simulink library "Lib_LongPRACH"  (R2023b)
settings: Solver=VariableStepAuto  StartTime=0.0  StopTime=10.0  RelTol=1e-3
values from neighbouring files (symbols this model uses):
  prach = waveconfig.PRACH.Config    [hNRPRACHWaveformGenerator.m]
undefined symbols (not defined in the file or in its folder): AdvDSPBChannelOutDisplay, AdvDSPBDMemDisplay, AdvDSPBInDisplay, AdvDSPBOutDisplay, dpoly, dspba, dspba_ChannelInVis, dspba_ChannelOutVis, dspba_internal_get_channel_ports, evalAionMaskParam, latency, latencyCorrection, NTxAnts, primtype, UseDontCare, value
libraries: DSPBAPrim x553, DSPBABase x32, DSPBAFilters x24, DSPBAControl x18, DSPBAModelBus x8, DSPBAWaveformSynth x4, DspbAdvFftLibrary x2, DSPBAUtilities x2
(part 4 of 8)

== system Lib_LongPRACH/prach_wrap/DECIMATION/Filt_DEC_by_2_stage3 ==
  din : Inport
  vin : Inport  Port=2
  cin : Inport  Port=3
  Complex to Real-Imag : ComplexToRealImag
  Const1 : DSPBAPrim/Const  primtype=const  nInputs=0  nOutputs=1  omode=Inherit via back propagation  otype=ufix(8)  scale=2^0  rndmethod=Unbiased  factor=1  satmethod=Symmetric  shift_vec=[0 1 2 -1]  value=deimator_shift  inPortNames=['+'; '+';]  outPortNames=[' ']  dspbaimage=dspba_prim.svg  text=fprintf('%s', num2str(value));  style=Optimised  visibilities=8 + 1024  floatPrecision=float32_m23  warnSaturation=on  version=20211007  SampleTime=inf
  Const6 : DSPBAPrim/Const  primtype=const  nInputs=0  nOutputs=1  omode=Inherit via back propagation  otype=ufix(8)  scale=2^0  rndmethod=Unbiased  factor=1  satmethod=Symmetric  shift_vec=[0 1 2 -1]  value=deimator_shift  inPortNames=['+'; '+';]  outPortNames=[' ']  dspbaimage=dspba_prim.svg  text=fprintf('%s', num2str(value));  style=Optimised  visibilities=8 + 1024  floatPrecision=float32_m23  warnSaturation=on  version=20211007  SampleTime=inf
  DecimatingFIR : DSPBAFilters/DecimatingFIR  nInputRate=prach.MaxSampleRate/(3*2)  decim=2  nchan=prach.no_of_chan  symmetry=Symmetrical  coef=b_decimator3  addr=MMoffset.HBcoef3  rwmode=Constant  nband=Use All Taps  exposebus=off  latency=46  version=20090407  recon=off  MM=[0,1,2,3,4,5,6,7,8,9,10,11,12,13,14,15]  resetrezero=off  sharecoef=auto  simulationMode=Standard
  DecimatingFIR1 : DSPBAFilters/DecimatingFIR  nInputRate=prach.MaxSampleRate/(3*2)  decim=2  nchan=prach.no_of_chan  symmetry=Symmetrical  coef=b_decimator3  addr=MMoffset.HBcoef3  rwmode=Constant  nband=Use All Taps  exposebus=off  latency=46  version=20090407  recon=off  MM=[0,1,2,3,4,5,6,7,8,9,10,11,12,13,14,15]  resetrezero=off  sharecoef=auto  simulationMode=Standard
  Real-Imag to Complex : RealImagToComplex
  Scale : DSPBABase/Scale  otype=sfix(16)  scale=2^-15  rndmethod=Biased  factor=decimator_gain3  satmethod=Symmetric  shift_vec=0  latency=5  simulationMode=Use Global Value  version=20130807
  Scale1 : DSPBABase/Scale  otype=sfix(16)  scale=2^-15  rndmethod=Biased  factor=decimator_gain3  satmethod=Symmetric  shift_vec=0  latency=5  simulationMode=Use Global Value  version=20130807
  Terminator{,1..3} (4 alike) : Terminator
  To Workspace3 : ToWorkspace  VariableName=dec_dout_stage3  SampleTime=-1
  To Workspace4 : ToWorkspace  VariableName=dec_vout_stage3  SampleTime=-1
  dout : Outport  VectorParamsAs1DForOutWhenUnconnected=off
  vout : Outport  Port=2  VectorParamsAs1DForOutWhenUnconnected=off
  cout : Outport  Port=3  VectorParamsAs1DForOutWhenUnconnected=off
  wires:
  DecimatingFIR/1 -> Scale/1
  Const6/1 -> Scale/4
  cin/1 -> DecimatingFIR1/3, DecimatingFIR/3
  Scale/4 -> Terminator/1
  DecimatingFIR/3 -> Scale/3
  vin/1 -> DecimatingFIR1/2, DecimatingFIR/2
  DecimatingFIR/2 -> Scale/2
  Scale/3 -> cout/1
  din/1 -> Complex to Real-Imag/1
  Complex to Real-Imag/1 -> DecimatingFIR/1
  Complex to Real-Imag/2 -> DecimatingFIR1/1
  DecimatingFIR1/1 -> Scale1/1
  DecimatingFIR1/3 -> Scale1/3
  Scale1/1 -> Real-Imag to Complex/2
  DecimatingFIR1/2 -> Scale1/2
  Const1/1 -> Scale1/4
  Scale1/4 -> Terminator1/1
  Scale/1 -> Real-Imag to Complex/1
  Scale1/2 -> Terminator2/1
  Scale1/3 -> Terminator3/1
  Scale/2 -> To Workspace4/1, vout/1
  Real-Imag to Complex/1 -> To Workspace3/1, dout/1

== system Lib_LongPRACH/prach_wrap/DECIMATION/Filt_DEC_by_2_stage4 ==
  din : Inport
  vin : Inport  Port=2
  cin : Inport  Port=3
  Complex to Real-Imag : ComplexToRealImag
  Const1 : DSPBAPrim/Const  primtype=const  nInputs=0  nOutputs=1  omode=Inherit via back propagation  otype=ufix(8)  scale=2^0  rndmethod=Unbiased  factor=1  satmethod=Symmetric  shift_vec=[0 1 2 -1]  value=deimator_shift  inPortNames=['+'; '+';]  outPortNames=[' ']  dspbaimage=dspba_prim.svg  text=fprintf('%s', num2str(value));  style=Optimised  visibilities=8 + 1024  floatPrecision=float32_m23  warnSaturation=on  version=20211007  SampleTime=inf
  Const6 : DSPBAPrim/Const  primtype=const  nInputs=0  nOutputs=1  omode=Inherit via back propagation  otype=ufix(8)  scale=2^0  rndmethod=Unbiased  factor=1  satmethod=Symmetric  shift_vec=[0 1 2 -1]  value=deimator_shift  inPortNames=['+'; '+';]  outPortNames=[' ']  dspbaimage=dspba_prim.svg  text=fprintf('%s', num2str(value));  style=Optimised  visibilities=8 + 1024  floatPrecision=float32_m23  warnSaturation=on  version=20211007  SampleTime=inf
  DecimatingFIR : DSPBAFilters/DecimatingFIR  nInputRate=prach.MaxSampleRate/(3*2*2)  decim=2  nchan=prach.no_of_chan  symmetry=Symmetrical  coef=b_decimator4  addr=MMoffset.HBcoef3  rwmode=Constant  nband=Use All Taps  exposebus=off  latency=98  version=20090407  recon=off  MM=[0,1,2,3,4,5,6,7,8,9,10,11,12,13,14,15]  resetrezero=off  sharecoef=auto  simulationMode=Standard
  DecimatingFIR1 : DSPBAFilters/DecimatingFIR  nInputRate=prach.MaxSampleRate/(3*2*2)  decim=2  nchan=prach.no_of_chan  symmetry=Symmetrical  coef=b_decimator4  addr=MMoffset.HBcoef3  rwmode=Constant  nband=Use All Taps  exposebus=off  latency=98  version=20090407  recon=off  MM=[0,1,2,3,4,5,6,7,8,9,10,11,12,13,14,15]  resetrezero=off  sharecoef=auto  simulationMode=Standard
  Real-Imag to Complex : RealImagToComplex
  Scale : DSPBABase/Scale  otype=sfix(16)  scale=2^-15  rndmethod=Biased  factor=decimator_gain4  satmethod=Symmetric  shift_vec=0  latency=5  simulationMode=Use Global Value  version=20130807
  Scale1 : DSPBABase/Scale  otype=sfix(16)  scale=2^-15  rndmethod=Biased  factor=decimator_gain4  satmethod=Symmetric  shift_vec=0  latency=5  simulationMode=Use Global Value  version=20130807
  Terminator{,1..3} (4 alike) : Terminator
  To Workspace3 : ToWorkspace  VariableName=dec_dout_stage4  SampleTime=-1
  To Workspace4 : ToWorkspace  VariableName=dec_vout_stage4  SampleTime=-1
  dout : Outport  VectorParamsAs1DForOutWhenUnconnected=off
  vout : Outport  Port=2  VectorParamsAs1DForOutWhenUnconnected=off
  cout : Outport  Port=3  VectorParamsAs1DForOutWhenUnconnected=off
  wires:
  DecimatingFIR/1 -> Scale/1
  Const6/1 -> Scale/4
  cin/1 -> DecimatingFIR1/3, DecimatingFIR/3
  Scale/4 -> Terminator/1
  DecimatingFIR/3 -> Scale/3
  vin/1 -> DecimatingFIR1/2, DecimatingFIR/2
  DecimatingFIR/2 -> Scale/2
  Scale/3 -> cout/1
  din/1 -> Complex to Real-Imag/1
  Complex to Real-Imag/1 -> DecimatingFIR/1
  Complex to Real-Imag/2 -> DecimatingFIR1/1
  DecimatingFIR1/1 -> Scale1/1
  DecimatingFIR1/3 -> Scale1/3
  Scale1/1 -> Real-Imag to Complex/2
  DecimatingFIR1/2 -> Scale1/2
  Const1/1 -> Scale1/4
  Scale1/4 -> Terminator1/1
  Scale/1 -> Real-Imag to Complex/1
  Scale1/2 -> Terminator2/1
  Scale1/3 -> Terminator3/1
  Scale/2 -> To Workspace4/1, vout/1
  Real-Imag to Complex/1 -> To Workspace3/1, dout/1

== system Lib_LongPRACH/prach_wrap/DECIMATION/Filt_DEC_by_2_stage5 ==
  din : Inport
  vin : Inport  Port=2
  cin : Inport  Port=3
  Complex to Real-Imag : ComplexToRealImag
  Const1 : DSPBAPrim/Const  primtype=const  nInputs=0  nOutputs=1  omode=Inherit via back propagation  otype=ufix(8)  scale=2^0  rndmethod=Unbiased  factor=1  satmethod=Symmetric  shift_vec=[0 1 2 -1]  value=deimator_shift  inPortNames=['+'; '+';]  outPortNames=[' ']  dspbaimage=dspba_prim.svg  text=fprintf('%s', num2str(value));  style=Optimised  visibilities=8 + 1024  floatPrecision=float32_m23  warnSaturation=on  version=20211007  SampleTime=inf
  Const6 : DSPBAPrim/Const  primtype=const  nInputs=0  nOutputs=1  omode=Inherit via back propagation  otype=ufix(8)  scale=2^0  rndmethod=Unbiased  factor=1  satmethod=Symmetric  shift_vec=[0 1 2 -1]  value=deimator_shift  inPortNames=['+'; '+';]  outPortNames=[' ']  dspbaimage=dspba_prim.svg  text=fprintf('%s', num2str(value));  style=Optimised  visibilities=8 + 1024  floatPrecision=float32_m23  warnSaturation=on  version=20211007  SampleTime=inf
  DecimatingFIR : DSPBAFilters/DecimatingFIR  nInputRate=prach.MaxSampleRate/(3*2*2*2)  decim=2  nchan=prach.no_of_chan  symmetry=Symmetrical  coef=b_decimator5  addr=MMoffset.HBcoef3  rwmode=Constant  nband=Use All Taps  exposebus=off  latency=176  version=20090407  recon=off  MM=[0,1,2,3,4,5,6,7,8,9,10,11,12,13,14,15]  resetrezero=off  sharecoef=auto  simulationMode=Standard
  DecimatingFIR1 : DSPBAFilters/DecimatingFIR  nInputRate=prach.MaxSampleRate/(3*2*2*2)  decim=2  nchan=prach.no_of_chan  symmetry=Symmetrical  coef=b_decimator5  addr=MMoffset.HBcoef3  rwmode=Constant  nband=Use All Taps  exposebus=off  latency=176  version=20090407  recon=off  MM=[0,1,2,3,4,5,6,7,8,9,10,11,12,13,14,15]  resetrezero=off  sharecoef=auto  simulationMode=Standard
  Real-Imag to Complex : RealImagToComplex
  Scale : DSPBABase/Scale  otype=sfix(16)  scale=2^-15  rndmethod=Biased  factor=decimator_gain5  satmethod=Symmetric  shift_vec=0  latency=5  simulationMode=Use Global Value  version=20130807
  Scale1 : DSPBABase/Scale  otype=sfix(16)  scale=2^-15  rndmethod=Biased  factor=decimator_gain5  satmethod=Symmetric  shift_vec=0  latency=5  simulationMode=Use Global Value  version=20130807
  Terminator{,1..3} (4 alike) : Terminator
  To Workspace3 : ToWorkspace  VariableName=dec_dout_stage5  SampleTime=-1
  To Workspace4 : ToWorkspace  VariableName=dec_vout_stage5  SampleTime=-1
  dout : Outport  VectorParamsAs1DForOutWhenUnconnected=off
  vout : Outport  Port=2  VectorParamsAs1DForOutWhenUnconnected=off
  cout : Outport  Port=3  VectorParamsAs1DForOutWhenUnconnected=off
  wires:
  DecimatingFIR/1 -> Scale/1
  Const6/1 -> Scale/4
  cin/1 -> DecimatingFIR1/3, DecimatingFIR/3
  Scale/4 -> Terminator/1
  DecimatingFIR/3 -> Scale/3
  vin/1 -> DecimatingFIR1/2, DecimatingFIR/2
  DecimatingFIR/2 -> Scale/2
  Scale/3 -> cout/1
  din/1 -> Complex to Real-Imag/1
  Complex to Real-Imag/1 -> DecimatingFIR/1
  Complex to Real-Imag/2 -> DecimatingFIR1/1
  DecimatingFIR1/1 -> Scale1/1
  DecimatingFIR1/3 -> Scale1/3
  Scale1/1 -> Real-Imag to Complex/2
  DecimatingFIR1/2 -> Scale1/2
  Const1/1 -> Scale1/4
  Scale1/4 -> Terminator1/1
  Scale/1 -> Real-Imag to Complex/1
  Scale1/2 -> Terminator2/1
  Scale1/3 -> Terminator3/1
  Scale/2 -> vout/1, To Workspace4/1
  Real-Imag to Complex/1 -> dout/1, To Workspace3/1

== system Lib_LongPRACH/prach_wrap/DECIMATION/Filt_DEC_by_2_stage6 ==
  din : Inport
  vin : Inport  Port=2
  cin : Inport  Port=3
  Complex to Real-Imag : ComplexToRealImag
  Const1 : DSPBAPrim/Const  primtype=const  nInputs=0  nOutputs=1  omode=Inherit via back propagation  otype=ufix(8)  scale=2^0  rndmethod=Unbiased  factor=1  satmethod=Symmetric  shift_vec=[0 1 2 -1]  value=deimator_shift  inPortNames=['+'; '+';]  outPortNames=[' ']  dspbaimage=dspba_prim.svg  text=fprintf('%s', num2str(value));  style=Optimised  visibilities=8 + 1024  floatPrecision=float32_m23  warnSaturation=on  version=20211007  SampleTime=inf
  Const6 : DSPBAPrim/Const  primtype=const  nInputs=0  nOutputs=1  omode=Inherit via back propagation  otype=ufix(8)  scale=2^0  rndmethod=Unbiased  factor=1  satmethod=Symmetric  shift_vec=[0 1 2 -1]  value=deimator_shift  inPortNames=['+'; '+';]  outPortNames=[' ']  dspbaimage=dspba_prim.svg  text=fprintf('%s', num2str(value));  style=Optimised  visibilities=8 + 1024  floatPrecision=float32_m23  warnSaturation=on  version=20211007  SampleTime=inf
  DecimatingFIR : DSPBAFilters/DecimatingFIR  nInputRate=prach.MaxSampleRate/(3*2*2*2*2)  decim=2  nchan=prach.no_of_chan  symmetry=Symmetrical  coef=b_decimator6  addr=MMoffset.HBcoef3  rwmode=Constant  nband=Use All Taps  exposebus=off  latency=208  version=20090407  recon=off  MM=[0,1,2,3,4,5,6,7,8,9,10,11,12,13,14,15]  resetrezero=off  sharecoef=auto  simulationMode=Standard
  DecimatingFIR1 : DSPBAFilters/DecimatingFIR  nInputRate=prach.MaxSampleRate/(3*2*2*2*2)  decim=2  nchan=prach.no_of_chan  symmetry=Symmetrical  coef=b_decimator6  addr=MMoffset.HBcoef3  rwmode=Constant  nband=Use All Taps  exposebus=off  latency=208  version=20090407  recon=off  MM=[0,1,2,3,4,5,6,7,8,9,10,11,12,13,14,15]  resetrezero=off  sharecoef=auto  simulationMode=Standard
  Real-Imag to Complex : RealImagToComplex
  Scale : DSPBABase/Scale  otype=sfix(16)  scale=2^-15  rndmethod=Biased  factor=decimator_gain6  satmethod=Symmetric  shift_vec=0  latency=5  simulationMode=Use Global Value  version=20130807
  Scale1 : DSPBABase/Scale  otype=sfix(16)  scale=2^-15  rndmethod=Biased  factor=decimator_gain6  satmethod=Symmetric  shift_vec=0  latency=5  simulationMode=Use Global Value  version=20130807
  Terminator{,1..3} (4 alike) : Terminator
  dout : Outport  VectorParamsAs1DForOutWhenUnconnected=off
  vout : Outport  Port=2  VectorParamsAs1DForOutWhenUnconnected=off
  cout : Outport  Port=3  VectorParamsAs1DForOutWhenUnconnected=off
  wires:
  DecimatingFIR/1 -> Scale/1
  Const6/1 -> Scale/4
  cin/1 -> DecimatingFIR1/3, DecimatingFIR/3
  Scale/4 -> Terminator/1
  Scale/2 -> vout/1
  DecimatingFIR/3 -> Scale/3
  vin/1 -> DecimatingFIR1/2, DecimatingFIR/2
  DecimatingFIR/2 -> Scale/2
  Scale/3 -> cout/1
  din/1 -> Complex to Real-Imag/1
  Complex to Real-Imag/1 -> DecimatingFIR/1
  Complex to Real-Imag/2 -> DecimatingFIR1/1
  DecimatingFIR1/1 -> Scale1/1
  DecimatingFIR1/3 -> Scale1/3
  Scale1/1 -> Real-Imag to Complex/2
  DecimatingFIR1/2 -> Scale1/2
  Const1/1 -> Scale1/4
  Scale1/4 -> Terminator1/1
  Scale/1 -> Real-Imag to Complex/1
  Real-Imag to Complex/1 -> dout/1
  Scale1/2 -> Terminator2/1
  Scale1/3 -> Terminator3/1

== system Lib_LongPRACH/prach_wrap/DECIMATION/Filt_DEC_by_3_stage1 ==
  din : Inport
  vin : Inport  Port=2
  cin : Inport  Port=3
  Complex to Real-Imag : ComplexToRealImag
  Const1 : DSPBAPrim/Const  primtype=const  nInputs=0  nOutputs=1  omode=Inherit via back propagation  otype=ufix(8)  scale=2^0  rndmethod=Unbiased  factor=1  satmethod=Symmetric  shift_vec=[0 1 2 -1]  value=deimator_shift  inPortNames=['+'; '+';]  outPortNames=[' ']  dspbaimage=dspba_prim.svg  text=fprintf('%s', num2str(value));  style=Optimised  visibilities=8 + 1024  floatPrecision=float32_m23  warnSaturation=on  version=20211007  SampleTime=inf
  Const6 : DSPBAPrim/Const  primtype=const  nInputs=0  nOutputs=1  omode=Inherit via back propagation  otype=ufix(8)  scale=2^0  rndmethod=Unbiased  factor=1  satmethod=Symmetric  shift_vec=[0 1 2 -1]  value=deimator_shift  inPortNames=['+'; '+';]  outPortNames=[' ']  dspbaimage=dspba_prim.svg  text=fprintf('%s', num2str(value));  style=Optimised  visibilities=8 + 1024  floatPrecision=float32_m23  warnSaturation=on  version=20211007  SampleTime=inf
  DecimatingFIR1 : DSPBAFilters/DecimatingFIR  nInputRate=prach.MaxSampleRate  decim=3  nchan=prach.no_of_chan  symmetry=Symmetrical  coef=b_decimator1  addr=MMoffset.decby3_st2  rwmode=Constant  nband=Use All Taps  exposebus=off  latency=26  version=20090407  recon=off  MM=[0,1,2,3,4,5,6,7,8,9,10,11,12,13,14,15]  resetrezero=off  sharecoef=auto  simulationMode=Standard
  DecimatingFIR2 : DSPBAFilters/DecimatingFIR  nInputRate=prach.MaxSampleRate  decim=3  nchan=prach.no_of_chan  symmetry=Symmetrical  coef=b_decimator1  addr=MMoffset.decby3_st2  rwmode=Constant  nband=Use All Taps  exposebus=off  latency=26  version=20090407  recon=off  MM=[0,1,2,3,4,5,6,7,8,9,10,11,12,13,14,15]  resetrezero=off  sharecoef=auto  simulationMode=Standard
  Real-Imag to Complex : RealImagToComplex
  Scale : DSPBABase/Scale  otype=sfix(16)  scale=2^-15  rndmethod=Biased  factor=decimator_gain1  satmethod=Symmetric  shift_vec=0  latency=5  simulationMode=Use Global Value  version=20130807
  Scale1 : DSPBABase/Scale  otype=sfix(16)  scale=2^-15  rndmethod=Biased  factor=decimator_gain1  satmethod=Symmetric  shift_vec=0  latency=5  simulationMode=Use Global Value  version=20130807
  Terminator : Terminator
  Terminator1 : Terminator
  To Workspace3 : ToWorkspace  VariableName=dec_dout_stage1  SampleTime=-1
  To Workspace4 : ToWorkspace  VariableName=dec_vout_stage1  SampleTime=-1
  dout : Outport  VectorParamsAs1DForOutWhenUnconnected=off
  vout : Outport  Port=2  VectorParamsAs1DForOutWhenUnconnected=off
  cout : Outport  Port=3  VectorParamsAs1DForOutWhenUnconnected=off
  wires:
  Scale/3 -> cout/1
  DecimatingFIR2/2 -> Scale/2
  vin/1 -> DecimatingFIR1/2, DecimatingFIR2/2
  DecimatingFIR2/3 -> Scale/3
  Scale/2 -> To Workspace4/1, vout/1
  Scale/4 -> Terminator/1
  cin/1 -> DecimatingFIR1/3, DecimatingFIR2/3
  Const6/1 -> Scale/4
  DecimatingFIR2/1 -> Scale/1
  din/1 -> Complex to Real-Imag/1
  Complex to Real-Imag/1 -> DecimatingFIR2/1
  Complex to Real-Imag/2 -> DecimatingFIR1/1
  Scale1/1 -> Real-Imag to Complex/2
  DecimatingFIR1/3 -> Scale1/3
  Scale1/4 -> Terminator1/1
  DecimatingFIR1/1 -> Scale1/1
  DecimatingFIR1/2 -> Scale1/2
  Const1/1 -> Scale1/4
  Real-Imag to Complex/1 -> To Workspace3/1, dout/1
  Scale/1 -> Real-Imag to Complex/1

== system Lib_LongPRACH/prach_wrap/FFTShift/ChNoLatch ==
  valid1 : Inport
  din : Inport  Port=2
  valid2 : Inport  Port=3
  FIFO : DSPBAPrim/FIFO  primtype=fifo  nInputs=3  nOutputs=4  omode=Inherit via internal rule  otype=sfix(16)  scale=2^-15  rndmethod=Unbiased  factor=1  satmethod=Symmetric  shift_vec=[0 1 2 -1]  value=[32 4 16]  inPortNames=['w'; 'd'; 'r'; 'f']  outPortNames=['v'; 'q'; 't'; 'f']  dspbaimage=dspba_prim_tall.svg  text=fprintf('fifo');  style=Optimised  visibilities=263168  version=20211007  user_sclr=off
  Terminator1 : Terminator
  Terminator2 : Terminator
  Terminator3 : Terminator
  risingedge : Subsystem
  risingedge1 : Subsystem
  dout : Outport
  wires:
  FIFO/3 -> Terminator1/1
  FIFO/1 -> Terminator3/1
  risingedge1/1(Out1) -> FIFO/3
  FIFO/4 -> Terminator2/1
  risingedge/1(Out1) -> FIFO/1
  valid2/1 -> risingedge1/1(In2)
  FIFO/2 -> dout/1
  valid1/1 -> risingedge/1(In2)
  din/1 -> FIFO/2

== system Lib_LongPRACH/prach_wrap/FFTShift/Mem_rd_wr ==
  valid : Inport
  Mem_rd_control : Subsystem
  Mem_wr_control : Subsystem
  Wr_addr_final : Outport
  We : Outport  Port=2
  rd_addr_final : Outport  Port=3
  rd_validout : Outport  Port=4
  wba : Outport  Port=5
  wires:
  valid/1 -> Mem_wr_control/1(valid)
  Mem_wr_control/1(wr_addr_final) -> Wr_addr_final/1
  Mem_wr_control/2(we) -> We/1
  Mem_wr_control/3(wba) -> wba/1, Mem_rd_control/1(wba)
  Mem_rd_control/1(rd_addr_final) -> rd_addr_final/1
  Mem_rd_control/2(validout) -> rd_validout/1

== system Lib_LongPRACH/prach_wrap/FFTShift/Subsystem ==
  toggleline : Inport
  d : Inport  Port=2
  SampleDelay : DSPBAPrim/SampleDelay  primtype=sampdelay  nInputs=1  nOutputs=1  omode=Inherit via internal rule  otype=sfix(16)  scale=2^-15  rndmethod=Unbiased  factor=1  satmethod=Symmetric  shift_vec=[0 1 2 -1]  floatPrecision=float32_m23  value=1  inPortNames=[' '; ' ';]  outPortNames=[' ']  dspbaimage=dspba_prim.svg  text=dpoly(1, eye(1,value+1), 'z')  style=Optimised  visibilities=8 + 2^11 + 2^18 + 2^19  flexible=off  slackgroup=0  augmented=0  version=20211007  advOptions=[]
  Xor : DSPBAPrim/Xor  primtype=xor  nInputs=2  nOutputs=1  omode=Inherit via internal rule  otype=sfix(16)  scale=2^-15  rndmethod=Unbiased  factor=1  satmethod=Symmetric  shift_vec=[0 1 2 -1]  value=0  inPortNames=[' '; ' '; ' '; ' '; ' '; ' '; ' '; ' '; ' '; ' '; ' '; ' '; ' '; ' '; ' '; ' '; ]  outPortNames=[' ']  dspbaimage=dspba_prim.svg  text=fprintf('^');  style=Optimised  visibilities=8+2  version=20211007
  latch_0L : DSPBAControl/latch_0L
  q : Outport
  wires:
  SampleDelay/1 -> Xor/1
  Xor/1 -> latch_0L/1
  latch_0L/1 -> q/1
  d/1 -> latch_0L/2
  toggleline/1 -> SampleDelay/1, Xor/2

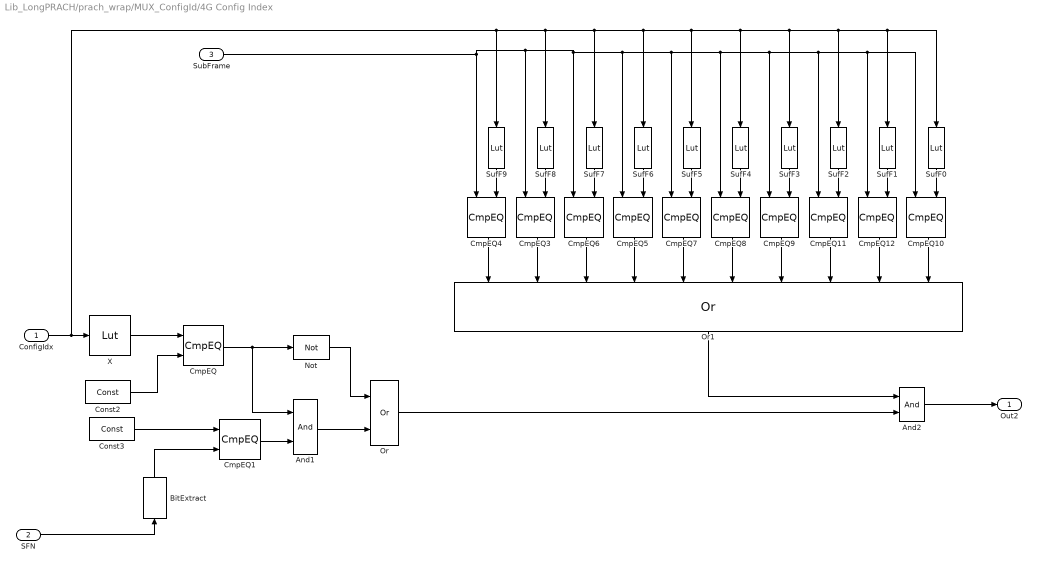
== system Lib_LongPRACH/prach_wrap/MUX_ConfigId/4G Config Index ==
  ConfigIdx : Inport
  SFN : Inport  Port=2
  SubFrame : Inport  Port=3
  And1 : DSPBAPrim/And  primtype=and  nInputs=2  nOutputs=1  omode=Inherit via internal rule  otype=sfix(16)  scale=2^-15  rndmethod=Unbiased  factor=1  satmethod=Symmetric  shift_vec=[0 1 2 -1]  value=0  inPortNames=[' '; ' '; ' '; ' '; ' '; ' '; ' '; ' '; ' '; ' '; ' '; ' '; ' '; ' '; ' '; ' '; ]  outPortNames=[' ']  dspbaimage=dspba_prim.svg  text=fprintf('&');  style=Optimised  visibilities=8+2  version=20211007
  And2 : DSPBAPrim/And  primtype=and  nInputs=2  nOutputs=1  omode=Inherit via internal rule  otype=sfix(16)  scale=2^-15  rndmethod=Unbiased  factor=1  satmethod=Symmetric  shift_vec=[0 1 2 -1]  value=0  inPortNames=[' '; ' '; ' '; ' '; ' '; ' '; ' '; ' '; ' '; ' '; ' '; ' '; ' '; ' '; ' '; ' '; ]  outPortNames=[' ']  dspbaimage=dspba_prim.svg  text=fprintf('&');  style=Optimised  visibilities=8+2  version=20211007
  BitExtract : DSPBAPrim/BitExtract  primtype=bitextract  nInputs=1  nOutputs=1  omode=Specify via dialog  otype=ufix(1)  scale=1  rndmethod=Unbiased  factor=1  satmethod=Symmetric  shift_vec=[0 1 2 -1]  value=0  inPortNames=[' '; ' ';]  outPortNames=[' ']  dspbaimage=dspba_prim.svg  text=fprintf('..%d', value);  style=Optimised  visibilities=8+1024  version=20211007
  CmpEQ{,1,3..12} (12 alike) : DSPBAPrim/CmpEQ  primtype=cmpeq  nInputs=2  nOutputs=1  omode=boolean  otype=sfix(16)  scale=2^-15  rndmethod=Unbiased  factor=1  satmethod=Symmetric  shift_vec=[0 1 2 -1]  value=0  inPortNames=[' '; ' ';]  outPortNames=[' ']  dspbaimage=dspba_prim.svg  text=fprintf('==');  style=Optimised  visibilities=0  advOptions=[]  version=20211007
  Const2 : DSPBAPrim/Const  primtype=const  nInputs=0  nOutputs=1  omode=Specify via dialog  otype=ufix(1)  scale=2^-0  rndmethod=Unbiased  factor=1  satmethod=Symmetric  shift_vec=[0 1 2 -1]  value=0  inPortNames=['+'; '+';]  outPortNames=[' ']  dspbaimage=dspba_prim.svg  text=fprintf('%s', num2str(value));  style=Optimised  visibilities=8 + 1024  floatPrecision=float32_m23  warnSaturation=on  version=20211007  SampleTime=inf
  Const3 : DSPBAPrim/Const  primtype=const  nInputs=0  nOutputs=1  omode=Specify via dialog  otype=ufix(1)  scale=2^-0  rndmethod=Unbiased  factor=1  satmethod=Symmetric  shift_vec=[0 1 2 -1]  value=0  inPortNames=['+'; '+';]  outPortNames=[' ']  dspbaimage=dspba_prim.svg  text=fprintf('%s', num2str(value));  style=Optimised  visibilities=8 + 1024  floatPrecision=float32_m23  warnSaturation=on  version=20211007  SampleTime=inf
  Not : DSPBAPrim/Not  primtype=not  nInputs=1  nOutputs=1  omode=Inherit via internal rule  otype=sfix(16)  scale=2^-15  rndmethod=Unbiased  factor=1  satmethod=Symmetric  shift_vec=[0 1 2 -1]  value=0  inPortNames=[' '; ' ';]  outPortNames=[' ']  dspbaimage=dspba_prim.svg  text=fprintf('~');  style=Optimised  visibilities=8  version=20211007
  Or : DSPBAPrim/Or  primtype=or  nInputs=2  nOutputs=1  omode=Inherit via internal rule  otype=sfix(16)  scale=2^-15  rndmethod=Unbiased  factor=1  satmethod=Symmetric  shift_vec=[0 1 2 -1]  value=0  inPortNames=[' '; ' '; ' '; ' '; ' '; ' '; ' '; ' '; ' '; ' '; ' '; ' '; ' '; ' '; ' '; ' '; ]  outPortNames=[' ']  dspbaimage=dspba_prim.svg  text=fprintf('|');  style=Optimised  visibilities=8+2  version=20211007
  Or1 : DSPBAPrim/Or  primtype=or  nInputs=10  nOutputs=1  omode=Inherit via internal rule  otype=sfix(16)  scale=2^-15  rndmethod=Unbiased  factor=1  satmethod=Symmetric  shift_vec=[0 1 2 -1]  value=0  inPortNames=[' '; ' '; ' '; ' '; ' '; ' '; ' '; ' '; ' '; ' '; ' '; ' '; ' '; ' '; ' '; ' '; ]  outPortNames=[' ']  dspbaimage=dspba_prim.svg  text=fprintf('|');  style=Optimised  visibilities=8+2  version=20211007
  SufF0 : DSPBAPrim/Lut  primtype=lut  nInputs=1  nOutputs=1  omode=Inherit via internal rule  otype=sfix(16)  scale=2^-15  rndmethod=Unbiased  factor=1  satmethod=Symmetric  shift_vec=[0 1 2 -1]  value=[1 4 7 1 4 7 1 2 3 1 2 3 0 1 0 9 zeros(1,256-16)]  inPortNames=[' '; ' ';]  outPortNames=[' ']  dspbaimage=dspba_prim.svg  text=fprintf('LUT');  style=Optimised  visibilities=8 + 1024  floatPrecision=float32_m23  version=20211007
  SufF1 : DSPBAPrim/Lut  primtype=lut  nInputs=1  nOutputs=1  omode=Inherit via internal rule  otype=sfix(16)  scale=2^-15  rndmethod=Unbiased  factor=1  satmethod=Symmetric  shift_vec=[0 1 2 -1]  value=[1 4 7 1 4 7 6 7 8 4 5 6 2 3 1 9 zeros(1,256-16)]  inPortNames=[' '; ' ';]  outPortNames=[' ']  dspbaimage=dspba_prim.svg  text=fprintf('LUT');  style=Optimised  visibilities=8 + 1024  floatPrecision=float32_m23  version=20211007
  SufF2 : DSPBAPrim/Lut  primtype=lut  nInputs=1  nOutputs=1  omode=Inherit via internal rule  otype=sfix(16)  scale=2^-15  rndmethod=Unbiased  factor=1  satmethod=Symmetric  shift_vec=[0 1 2 -1]  value=[1 4 7 1 4 7 6 7 8 7 8 9 4 5 2 9 zeros(1,256-16)]  inPortNames=[' '; ' ';]  outPortNames=[' ']  dspbaimage=dspba_prim.svg  text=fprintf('LUT');  style=Optimised  visibilities=8 + 1024  floatPrecision=float32_m23  version=20211007
  SufF3 : DSPBAPrim/Lut  primtype=lut  nInputs=1  nOutputs=1  omode=Inherit via internal rule  otype=sfix(16)  scale=2^-15  rndmethod=Unbiased  factor=1  satmethod=Symmetric  shift_vec=[0 1 2 -1]  value=[1 4 7 1 4 7 6 7 8 7 8 9 6 7 3 9 zeros(1,256-16)]  inPortNames=[' '; ' ';]  outPortNames=[' ']  dspbaimage=dspba_prim.svg  text=fprintf('LUT');  style=Optimised  visibilities=8 + 1024  floatPrecision=float32_m23  version=20211007
  SufF4 : DSPBAPrim/Lut  primtype=lut  nInputs=1  nOutputs=1  omode=Inherit via internal rule  otype=sfix(16)  scale=2^-15  rndmethod=Unbiased  factor=1  satmethod=Symmetric  shift_vec=[0 1 2 -1]  value=[1 4 7 1 4 7 6 7 8 7 8 9 8 9 4 9 zeros(1,256-16)]  inPortNames=[' '; ' ';]  outPortNames=[' ']  dspbaimage=dspba_prim.svg  text=fprintf('LUT');  style=Optimised  visibilities=8 + 1024  floatPrecision=float32_m23  version=20211007
  SufF5 : DSPBAPrim/Lut  primtype=lut  nInputs=1  nOutputs=1  omode=Inherit via internal rule  otype=sfix(16)  scale=2^-15  rndmethod=Unbiased  factor=1  satmethod=Symmetric  shift_vec=[0 1 2 -1]  value=[1 4 7 1 4 7 6 7 8 7 8 9 8 9 5 9 zeros(1,256-16)]  inPortNames=[' '; ' ';]  outPortNames=[' ']  dspbaimage=dspba_prim.svg  text=fprintf('LUT');  style=Optimised  visibilities=8 + 1024  floatPrecision=float32_m23  version=20211007
  SufF6 : DSPBAPrim/Lut  primtype=lut  nInputs=1  nOutputs=1  omode=Inherit via internal rule  otype=sfix(16)  scale=2^-15  rndmethod=Unbiased  factor=1  satmethod=Symmetric  shift_vec=[0 1 2 -1]  value=[1 4 7 1 4 7 6 7 8 7 8 9 8 9 6 9 zeros(1,256-16)]  inPortNames=[' '; ' ';]  outPortNames=[' ']  dspbaimage=dspba_prim.svg  text=fprintf('LUT');  style=Optimised  visibilities=8 + 1024  floatPrecision=float32_m23  version=20211007
  SufF7 : DSPBAPrim/Lut  primtype=lut  nInputs=1  nOutputs=1  omode=Inherit via internal rule  otype=sfix(16)  scale=2^-15  rndmethod=Unbiased  factor=1  satmethod=Symmetric  shift_vec=[0 1 2 -1]  value=[1 4 7 1 4 7 6 7 8 7 8 9 8 9 7 9 zeros(1,256-16)]  inPortNames=[' '; ' ';]  outPortNames=[' ']  dspbaimage=dspba_prim.svg  text=fprintf('LUT');  style=Optimised  visibilities=8 + 1024  floatPrecision=float32_m23  version=20211007
  SufF8 : DSPBAPrim/Lut  primtype=lut  nInputs=1  nOutputs=1  omode=Inherit via internal rule  otype=sfix(16)  scale=2^-15  rndmethod=Unbiased  factor=1  satmethod=Symmetric  shift_vec=[0 1 2 -1]  value=[1 4 7 1 4 7 6 7 8 7 8 9 8 9 8 9 zeros(1,256-16)]  inPortNames=[' '; ' ';]  outPortNames=[' ']  dspbaimage=dspba_prim.svg  text=fprintf('LUT');  style=Optimised  visibilities=8 + 1024  floatPrecision=float32_m23  version=20211007
  SufF9 : DSPBAPrim/Lut  primtype=lut  nInputs=1  nOutputs=1  omode=Inherit via internal rule  otype=sfix(16)  scale=2^-15  rndmethod=Unbiased  factor=1  satmethod=Symmetric  shift_vec=[0 1 2 -1]  value=[1 4 7 1 4 7 6 7 8 7 8 9 8 9 9 9 zeros(1,256-16)]  inPortNames=[' '; ' ';]  outPortNames=[' ']  dspbaimage=dspba_prim.svg  text=fprintf('LUT');  style=Optimised  visibilities=8 + 1024  floatPrecision=float32_m23  version=20211007
  X : DSPBAPrim/Lut  primtype=lut  nInputs=1  nOutputs=1  omode=Inherit via internal rule  otype=sfix(16)  scale=2^-15  rndmethod=Unbiased  factor=1  satmethod=Symmetric  shift_vec=[0 1 2 -1]  value=[0,0,0,1,1,1,1,1,1,1,1,1,1,1,1,0,ones(1,256-16)]  inPortNames=[' '; ' ';]  outPortNames=[' ']  dspbaimage=dspba_prim.svg  text=fprintf('LUT');  style=Optimised  visibilities=8 + 1024  floatPrecision=float32_m23  version=20211007
  Out2 : Outport
  wires:
  Const3/1 -> CmpEQ1/1
  CmpEQ/1 -> Not/1, And1/1
  CmpEQ1/1 -> And1/2
  Not/1 -> Or/1
  X/1 -> CmpEQ/1
  Const2/1 -> CmpEQ/2
  And1/1 -> Or/2
  BitExtract/1 -> CmpEQ1/2
  Or/1 -> And2/2
  SFN/1 -> BitExtract/1
  CmpEQ10/1 -> Or1/10
  CmpEQ3/1 -> Or1/2
  CmpEQ6/1 -> Or1/3
  SufF3/1 -> CmpEQ9/2
  CmpEQ11/1 -> Or1/8
  CmpEQ5/1 -> Or1/4
  CmpEQ8/1 -> Or1/6
  CmpEQ12/1 -> Or1/9
  CmpEQ9/1 -> Or1/7
  CmpEQ4/1 -> Or1/1
  SufF4/1 -> CmpEQ8/2
  Or1/1 -> And2/1
  SufF0/1 -> CmpEQ10/2
  SufF5/1 -> CmpEQ7/2
  CmpEQ7/1 -> Or1/5
  SufF9/1 -> CmpEQ4/2
  SufF1/1 -> CmpEQ12/2
  ConfigIdx/1 -> X/1, SufF9/1, SufF8/1, SufF7/1, SufF6/1, SufF5/1, SufF4/1, SufF3/1, SufF2/1, SufF1/1, SufF0/1
  SufF7/1 -> CmpEQ6/2
  SufF2/1 -> CmpEQ11/2
  And2/1 -> Out2/1
  SufF6/1 -> CmpEQ5/2
  SufF8/1 -> CmpEQ3/2
  SubFrame/1 -> CmpEQ4/1, CmpEQ3/1, CmpEQ10/1, CmpEQ12/1, CmpEQ11/1, CmpEQ9/1, CmpEQ8/1, CmpEQ7/1, CmpEQ5/1, CmpEQ6/1

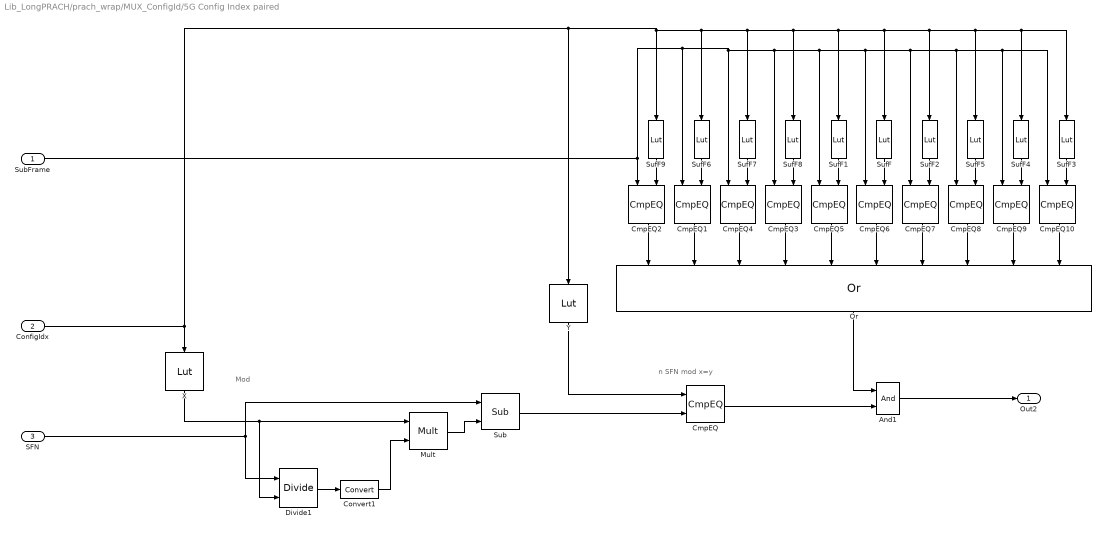
== system Lib_LongPRACH/prach_wrap/MUX_ConfigId/5G Config Index paired ==
  note: n SFN mod x=y
  note: Mod
  SubFrame : Inport
  ConfigIdx : Inport  Port=2
  SFN : Inport  Port=3
  And1 : DSPBAPrim/And  primtype=and  nInputs=2  nOutputs=1  omode=Inherit via internal rule  otype=sfix(16)  scale=2^-15  rndmethod=Unbiased  factor=1  satmethod=Symmetric  shift_vec=[0 1 2 -1]  value=0  inPortNames=[' '; ' '; ' '; ' '; ' '; ' '; ' '; ' '; ' '; ' '; ' '; ' '; ' '; ' '; ' '; ' '; ]  outPortNames=[' ']  dspbaimage=dspba_prim.svg  text=fprintf('&');  style=Optimised  visibilities=8+2  version=20211007
  CmpEQ{,1..10} (11 alike) : DSPBAPrim/CmpEQ  primtype=cmpeq  nInputs=2  nOutputs=1  omode=boolean  otype=sfix(16)  scale=2^-15  rndmethod=Unbiased  factor=1  satmethod=Symmetric  shift_vec=[0 1 2 -1]  value=0  inPortNames=[' '; ' ';]  outPortNames=[' ']  dspbaimage=dspba_prim.svg  text=fprintf('==');  style=Optimised  visibilities=0  advOptions=[]  version=20211007
  Convert1 : DSPBAPrim/Convert  primtype=convert  nInputs=1  nOutputs=1  omode=Specify via dialog  otype=uint(12)  scale=2^0  rndmethod=Truncate  factor=1  satmethod=None  shift_vec=[0 1 2 -1]  value=round([0:255]/17)  inPortNames=[' '; ' ';]  outPortNames=[' '; 'c']  dspbaimage=dspba_prim_wide.svg  text=fprintf('convert');  style=Optimised  visibilities=8+64+256+2^17  clipdetect=off  floatPrecision=float32_m23  advOptions=[]  version=20211007
  Divide1 : DSPBAPrim/Divide  primtype=divide  nInputs=2  nOutputs=1  omode=Inherit via internal rule  otype=ufix(4)  scale=2^-0  rndmethod=Unbiased  factor=1  satmethod=Symmetric  shift_vec=[0 1 2 -1]  value=round([0:255]/17)  inPortNames=[' '; ' ';]  outPortNames=[' ']  dspbaimage=dspba_prim.svg  text=fprintf('a\n----\nb');  style=Optimised  visibilities=8+2^17+2^18  floatRounding=correct  intDivider=off  advOptions=[]  version=20211007
  Mult : DSPBAPrim/Mult  primtype=mult  nInputs=2  nOutputs=1  omode=Inherit via internal rule  otype=sfix(16)  scale=2^-15  rndmethod=Unbiased  factor=1  satmethod=Symmetric  shift_vec=[0 1 2 -1]  value=0  inPortNames=[' '; ' ';]  outPortNames=[' ']  dspbaimage=dspba_prim.svg  text=fprintf('X');  style=Optimised  visibilities=8+2^18+2^19  floatPrecision=float32_m23  floatRounding=correct  advOptions=[]  version=20211007
  Or : DSPBAPrim/Or  primtype=or  nInputs=10  nOutputs=1  omode=Inherit via internal rule  otype=sfix(16)  scale=2^-15  rndmethod=Unbiased  factor=1  satmethod=Symmetric  shift_vec=[0 1 2 -1]  value=0  inPortNames=[' '; ' '; ' '; ' '; ' '; ' '; ' '; ' '; ' '; ' '; ' '; ' '; ' '; ' '; ' '; ' '; ]  outPortNames=[' ']  dspbaimage=dspba_prim.svg  text=fprintf('|');  style=Optimised  visibilities=8+2  version=20211007
  Sub : DSPBAPrim/Sub  primtype=sub  nInputs=2  nOutputs=1  omode=Specify via dialog  otype=uint(12)  scale=2^-0  rndmethod=Unbiased  factor=1  satmethod=Symmetric  shift_vec=[0 1 2 -1]  value=0  inPortNames=['+'; '-';]  outPortNames=[' ']  dspbaimage=dspba_prim.svg  text=fprintf('-');  style=Optimised  visibilities=8+2^17+2^18  floatRounding=correct  advOptions=[]  version=20211007
  SufF : DSPBAPrim/Lut  primtype=lut  nInputs=1  nOutputs=1  omode=Inherit via internal rule  otype=sfix(16)  scale=2^-15  rndmethod=Unbiased  factor=1  satmethod=Symmetric  shift_vec=[0 1 2 -1]  value=[1 4 7 9 1 4 7 9 1 4 7 9 1 4 7 9 1 4 7 1 2 3 1 2 3 0 1 5 zeros(1,256-28)]  inPortNames=[' '; ' ';]  outPortNames=[' ']  dspbaimage=dspba_prim.svg  text=fprintf('LUT');  style=Optimised  visibilities=8 + 1024  floatPrecision=float32_m23  version=20211007
  SufF1 : DSPBAPrim/Lut  primtype=lut  nInputs=1  nOutputs=1  omode=Inherit via internal rule  otype=sfix(16)  scale=2^-15  rndmethod=Unbiased  factor=1  satmethod=Symmetric  shift_vec=[0 1 2 -1]  value=[1 4 7 9 1 4 7 9 1 4 7 9 1 4 7 9 1 4 7 1 2 3 1 2 3 8 9 4 zeros(1,256-28)]  inPortNames=[' '; ' ';]  outPortNames=[' ']  dspbaimage=dspba_prim.svg  text=fprintf('LUT');  style=Optimised  visibilities=8 + 1024  floatPrecision=float32_m23  version=20211007
  SufF2 : DSPBAPrim/Lut  primtype=lut  nInputs=1  nOutputs=1  omode=Inherit via internal rule  otype=sfix(16)  scale=2^-15  rndmethod=Unbiased  factor=1  satmethod=Symmetric  shift_vec=[0 1 2 -1]  value=[1 4 7 9 1 4 7 9 1 4 7 9 1 4 7 9 1 4 7 1 2 3 1 2 3 0 1 6 zeros(1,256-28)]  inPortNames=[' '; ' ';]  outPortNames=[' ']  dspbaimage=dspba_prim.svg  text=fprintf('LUT');  style=Optimised  visibilities=8 + 1024  floatPrecision=float32_m23  version=20211007
  SufF3 : DSPBAPrim/Lut  primtype=lut  nInputs=1  nOutputs=1  omode=Inherit via internal rule  otype=sfix(16)  scale=2^-15  rndmethod=Unbiased  factor=1  satmethod=Symmetric  shift_vec=[0 1 2 -1]  value=[1 4 7 9 1 4 7 9 1 4 7 9 1 4 7 9 1 4 7 1 2 3 1 2 3 0 1 9 zeros(1,256-28)]  inPortNames=[' '; ' ';]  outPortNames=[' ']  dspbaimage=dspba_prim.svg  text=fprintf('LUT');  style=Optimised  visibilities=8 + 1024  floatPrecision=float32_m23  version=20211007
  SufF4 : DSPBAPrim/Lut  primtype=lut  nInputs=1  nOutputs=1  omode=Inherit via internal rule  otype=sfix(16)  scale=2^-15  rndmethod=Unbiased  factor=1  satmethod=Symmetric  shift_vec=[0 1 2 -1]  value=[1 4 7 9 1 4 7 9 1 4 7 9 1 4 7 9 1 4 7 1 2 3 1 2 3 0 1 8 zeros(1,256-28)]  inPortNames=[' '; ' ';]  outPortNames=[' ']  dspbaimage=dspba_prim.svg  text=fprintf('LUT');  style=Optimised  visibilities=8 + 1024  floatPrecision=float32_m23  version=20211007
  SufF5 : DSPBAPrim/Lut  primtype=lut  nInputs=1  nOutputs=1  omode=Inherit via internal rule  otype=sfix(16)  scale=2^-15  rndmethod=Unbiased  factor=1  satmethod=Symmetric  shift_vec=[0 1 2 -1]  value=[1 4 7 9 1 4 7 9 1 4 7 9 1 4 7 9 1 4 7 1 2 3 1 2 3 0 1 7 zeros(1,256-28)]  inPortNames=[' '; ' ';]  outPortNames=[' ']  dspbaimage=dspba_prim.svg  text=fprintf('LUT');  style=Optimised  visibilities=8 + 1024  floatPrecision=float32_m23  version=20211007
  SufF6 : DSPBAPrim/Lut  primtype=lut  nInputs=1  nOutputs=1  omode=Inherit via internal rule  otype=sfix(16)  scale=2^-15  rndmethod=Unbiased  factor=1  satmethod=Symmetric  shift_vec=[0 1 2 -1]  value=[1 4 7 9 1 4 7 9 1 4 7 9 1 4 7 9 1 4 7 1 2 3 1 2 3 0 1 0 zeros(1,256-28)]  inPortNames=[' '; ' ';]  outPortNames=[' ']  dspbaimage=dspba_prim.svg  text=fprintf('LUT');  style=Optimised  visibilities=8 + 1024  floatPrecision=float32_m23  version=20211007
  SufF7 : DSPBAPrim/Lut  primtype=lut  nInputs=1  nOutputs=1  omode=Inherit via internal rule  otype=sfix(16)  scale=2^-15  rndmethod=Unbiased  factor=1  satmethod=Symmetric  shift_vec=[0 1 2 -1]  value=[1 4 7 9 1 4 7 9 1 4 7 9 1 4 7 9 1 4 7 1 2 3 1 2 3 6 7 3 zeros(1,256-28)]  inPortNames=[' '; ' ';]  outPortNames=[' ']  dspbaimage=dspba_prim.svg  text=fprintf('LUT');  style=Optimised  visibilities=8 + 1024  floatPrecision=float32_m23  version=20211007
  SufF8 : DSPBAPrim/Lut  primtype=lut  nInputs=1  nOutputs=1  omode=Inherit via internal rule  otype=sfix(16)  scale=2^-15  rndmethod=Unbiased  factor=1  satmethod=Symmetric  shift_vec=[0 1 2 -1]  value=[1 4 7 9 1 4 7 9 1 4 7 9 1 4 7 9 1 4 7 1 2 3 7 8 9 4 5 2 zeros(1,256-28)]  inPortNames=[' '; ' ';]  outPortNames=[' ']  dspbaimage=dspba_prim.svg  text=fprintf('LUT');  style=Optimised  visibilities=8 + 1024  floatPrecision=float32_m23  version=20211007
  SufF9 : DSPBAPrim/Lut  primtype=lut  nInputs=1  nOutputs=1  omode=Inherit via internal rule  otype=sfix(16)  scale=2^-15  rndmethod=Unbiased  factor=1  satmethod=Symmetric  shift_vec=[0 1 2 -1]  value=[1 4 7 9 1 4 7 9 1 4 7 9 1 4 7 9 1 4 7 6 7 8 4 5 6 2 3 1 zeros(1,256-28)]  inPortNames=[' '; ' ';]  outPortNames=[' ']  dspbaimage=dspba_prim.svg  text=fprintf('LUT');  style=Optimised  visibilities=8 + 1024  floatPrecision=float32_m23  version=20211007
  X : DSPBAPrim/Lut  primtype=lut  nInputs=1  nOutputs=1  omode=Inherit via internal rule  otype=sfix(16)  scale=2^-15  rndmethod=Unbiased  factor=1  satmethod=Symmetric  shift_vec=[0 1 2 -1]  value=[16,16,16,16,8,8,8,8,4,4,4,4,2,2,2,2,1,1,1,1,1,1,1,1,1,1,1,1,ones(1,256-28)]  inPortNames=[' '; ' ';]  outPortNames=[' ']  dspbaimage=dspba_prim.svg  text=fprintf('LUT');  style=Optimised  visibilities=8 + 1024  floatPrecision=float32_m23  version=20211007
  Y : DSPBAPrim/Lut  primtype=lut  nInputs=1  nOutputs=1  omode=Inherit via internal rule  otype=sfix(16)  scale=2^-15  rndmethod=Unbiased  factor=1  satmethod=Symmetric  shift_vec=[0 1 2 -1]  value=[1 1 1 1 1 1 1 1 1 1 1 1 1 1 1 1 0 0 0 0 0 0 0 0 0 0 0 0 zeros(1,256-28)]  inPortNames=[' '; ' ';]  outPortNames=[' ']  dspbaimage=dspba_prim.svg  text=fprintf('LUT');  style=Optimised  visibilities=8 + 1024  floatPrecision=float32_m23  version=20211007
  Out2 : Outport
  wires:
  SufF5/1 -> CmpEQ8/2
  SubFrame/1 -> CmpEQ2/1, CmpEQ1/1, CmpEQ10/1, CmpEQ9/1, CmpEQ8/1, CmpEQ7/1, CmpEQ6/1, CmpEQ5/1, CmpEQ3/1, CmpEQ4/1
  X/1 -> Mult/1, Divide1/2
  ConfigIdx/1 -> SufF8/1, SufF3/1, SufF4/1, SufF5/1, SufF2/1, SufF/1, SufF1/1, SufF7/1, SufF6/1, SufF9/1, Y/1, X/1
  SufF1/1 -> CmpEQ5/2
  Divide1/1 -> Convert1/1
  SufF4/1 -> CmpEQ9/2
  SufF6/1 -> CmpEQ1/2
  SufF7/1 -> CmpEQ4/2
  CmpEQ5/1 -> Or/5
  Convert1/1 -> Mult/2
  CmpEQ/1 -> And1/2
  Or/1 -> And1/1
  CmpEQ2/1 -> Or/1
  SFN/1 -> Sub/1, Divide1/1
  SufF3/1 -> CmpEQ10/2
  Sub/1 -> CmpEQ/2
  Mult/1 -> Sub/2
  CmpEQ7/1 -> Or/7
  SufF8/1 -> CmpEQ3/2
  Y/1 -> CmpEQ/1
  CmpEQ9/1 -> Or/9
  CmpEQ6/1 -> Or/6
  CmpEQ8/1 -> Or/8
  CmpEQ3/1 -> Or/4
  CmpEQ1/1 -> Or/2
  CmpEQ4/1 -> Or/3
  SufF/1 -> CmpEQ6/2
  SufF2/1 -> CmpEQ7/2
  CmpEQ10/1 -> Or/10
  SufF9/1 -> CmpEQ2/2
  And1/1 -> Out2/1

== system Lib_LongPRACH/prach_wrap/MUX_ConfigId/5G Config Index unpaired ==
  note: n SFN mod x=y
  note: Mod
  SubFrame : Inport
  ConfigIdx : Inport  Port=2
  SFN : Inport  Port=3
  And1 : DSPBAPrim/And  primtype=and  nInputs=2  nOutputs=1  omode=Inherit via internal rule  otype=sfix(16)  scale=2^-15  rndmethod=Unbiased  factor=1  satmethod=Symmetric  shift_vec=[0 1 2 -1]  value=0  inPortNames=[' '; ' '; ' '; ' '; ' '; ' '; ' '; ' '; ' '; ' '; ' '; ' '; ' '; ' '; ' '; ' '; ]  outPortNames=[' ']  dspbaimage=dspba_prim.svg  text=fprintf('&');  style=Optimised  visibilities=8+2  version=20211007
  CmpEQ{,1..5} (6 alike) : DSPBAPrim/CmpEQ  primtype=cmpeq  nInputs=2  nOutputs=1  omode=boolean  otype=sfix(16)  scale=2^-15  rndmethod=Unbiased  factor=1  satmethod=Symmetric  shift_vec=[0 1 2 -1]  value=0  inPortNames=[' '; ' ';]  outPortNames=[' ']  dspbaimage=dspba_prim.svg  text=fprintf('==');  style=Optimised  visibilities=0  advOptions=[]  version=20211007
  Convert1 : DSPBAPrim/Convert  primtype=convert  nInputs=1  nOutputs=1  omode=Specify via dialog  otype=uint(12)  scale=2^0  rndmethod=Truncate  factor=1  satmethod=None  shift_vec=[0 1 2 -1]  value=round([0:255]/17)  inPortNames=[' '; ' ';]  outPortNames=[' '; 'c']  dspbaimage=dspba_prim_wide.svg  text=fprintf('convert');  style=Optimised  visibilities=8+64+256+2^17  clipdetect=off  floatPrecision=float32_m23  advOptions=[]  version=20211007
  Divide1 : DSPBAPrim/Divide  primtype=divide  nInputs=2  nOutputs=1  omode=Inherit via internal rule  otype=ufix(4)  scale=2^-0  rndmethod=Unbiased  factor=1  satmethod=Symmetric  shift_vec=[0 1 2 -1]  value=round([0:255]/17)  inPortNames=[' '; ' ';]  outPortNames=[' ']  dspbaimage=dspba_prim.svg  text=fprintf('a\n----\nb');  style=Optimised  visibilities=8+2^17+2^18  floatRounding=correct  intDivider=off  advOptions=[]  version=20211007
  Mult : DSPBAPrim/Mult  primtype=mult  nInputs=2  nOutputs=1  omode=Inherit via internal rule  otype=sfix(16)  scale=2^-15  rndmethod=Unbiased  factor=1  satmethod=Symmetric  shift_vec=[0 1 2 -1]  value=0  inPortNames=[' '; ' ';]  outPortNames=[' ']  dspbaimage=dspba_prim.svg  text=fprintf('X');  style=Optimised  visibilities=8+2^18+2^19  floatPrecision=float32_m23  floatRounding=correct  advOptions=[]  version=20211007
  Or : DSPBAPrim/Or  primtype=or  nInputs=5  nOutputs=1  omode=Inherit via internal rule  otype=sfix(16)  scale=2^-15  rndmethod=Unbiased  factor=1  satmethod=Symmetric  shift_vec=[0 1 2 -1]  value=0  inPortNames=[' '; ' '; ' '; ' '; ' '; ' '; ' '; ' '; ' '; ' '; ' '; ' '; ' '; ' '; ' '; ' '; ]  outPortNames=[' ']  dspbaimage=dspba_prim.svg  text=fprintf('|');  style=Optimised  visibilities=8+2  version=20211007
  Sub : DSPBAPrim/Sub  primtype=sub  nInputs=2  nOutputs=1  omode=Specify via dialog  otype=uint(12)  scale=2^-0  rndmethod=Unbiased  factor=1  satmethod=Symmetric  shift_vec=[0 1 2 -1]  value=0  inPortNames=['+'; '-';]  outPortNames=[' ']  dspbaimage=dspba_prim.svg  text=fprintf('-');  style=Optimised  visibilities=8+2^17+2^18  floatRounding=correct  advOptions=[]  version=20211007
  SufF1 : DSPBAPrim/Lut  primtype=lut  nInputs=1  nOutputs=1  omode=Inherit via internal rule  otype=sfix(16)  scale=2^-15  rndmethod=Unbiased  factor=1  satmethod=Symmetric  shift_vec=[0 1 2 -1]  value=Map_5g_LUT5  inPortNames=[' '; ' ';]  outPortNames=[' ']  dspbaimage=dspba_prim.svg  text=fprintf('LUT');  style=Optimised  visibilities=8 + 1024  floatPrecision=float32_m23  version=20211007
  SufF6 : DSPBAPrim/Lut  primtype=lut  nInputs=1  nOutputs=1  omode=Inherit via internal rule  otype=sfix(16)  scale=2^-15  rndmethod=Unbiased  factor=1  satmethod=Symmetric  shift_vec=[0 1 2 -1]  value=Map_5g_LUT2  inPortNames=[' '; ' ';]  outPortNames=[' ']  dspbaimage=dspba_prim.svg  text=fprintf('LUT');  style=Optimised  visibilities=8 + 1024  floatPrecision=float32_m23  version=20211007
  SufF7 : DSPBAPrim/Lut  primtype=lut  nInputs=1  nOutputs=1  omode=Inherit via internal rule  otype=sfix(16)  scale=2^-15  rndmethod=Unbiased  factor=1  satmethod=Symmetric  shift_vec=[0 1 2 -1]  value=Map_5g_LUT3  inPortNames=[' '; ' ';]  outPortNames=[' ']  dspbaimage=dspba_prim.svg  text=fprintf('LUT');  style=Optimised  visibilities=8 + 1024  floatPrecision=float32_m23  version=20211007
  SufF8 : DSPBAPrim/Lut  primtype=lut  nInputs=1  nOutputs=1  omode=Inherit via internal rule  otype=sfix(16)  scale=2^-15  rndmethod=Unbiased  factor=1  satmethod=Symmetric  shift_vec=[0 1 2 -1]  value=Map_5g_LUT4  inPortNames=[' '; ' ';]  outPortNames=[' ']  dspbaimage=dspba_prim.svg  text=fprintf('LUT');  style=Optimised  visibilities=8 + 1024  floatPrecision=float32_m23  version=20211007
  SufF9 : DSPBAPrim/Lut  primtype=lut  nInputs=1  nOutputs=1  omode=Inherit via internal rule  otype=sfix(16)  scale=2^-15  rndmethod=Unbiased  factor=1  satmethod=Symmetric  shift_vec=[0 1 2 -1]  value=Map_5g_LUT1  inPortNames=[' '; ' ';]  outPortNames=[' ']  dspbaimage=dspba_prim.svg  text=fprintf('LUT');  style=Optimised  visibilities=8 + 1024  floatPrecision=float32_m23  version=20211007
  X : DSPBAPrim/Lut  primtype=lut  nInputs=1  nOutputs=1  omode=Inherit via internal rule  otype=sfix(16)  scale=2^-15  rndmethod=Unbiased  factor=1  satmethod=Symmetric  shift_vec=[0 1 2 -1]  value=[16,16,16,16,8,8,8,8,4,4,4,4,2,2,2,2,1,1,1,1,1,1,1,1,1,1,1,1,ones(1,256-28)]  inPortNames=[' '; ' ';]  outPortNames=[' ']  dspbaimage=dspba_prim.svg  text=fprintf('LUT');  style=Optimised  visibilities=8 + 1024  floatPrecision=float32_m23  version=20211007
  Y : DSPBAPrim/Lut  primtype=lut  nInputs=1  nOutputs=1  omode=Inherit via internal rule  otype=sfix(16)  scale=2^-15  rndmethod=Unbiased  factor=1  satmethod=Symmetric  shift_vec=[0 1 2 -1]  value=[1 1 1 1 1 1 1 1 1 1 1 1 1 1 1 1 0 0 0 0 0 0 0 0 0 0 0 0 zeros(1,256-28)]  inPortNames=[' '; ' ';]  outPortNames=[' ']  dspbaimage=dspba_prim.svg  text=fprintf('LUT');  style=Optimised  visibilities=8 + 1024  floatPrecision=float32_m23  version=20211007
  Out2 : Outport
  wires:
  SubFrame/1 -> CmpEQ2/1, CmpEQ1/1, CmpEQ5/1, CmpEQ3/1, CmpEQ4/1
  X/1 -> Mult/1, Divide1/2
  ConfigIdx/1 -> SufF8/1, SufF1/1, SufF7/1, SufF6/1, SufF9/1, Y/1, X/1
  SufF1/1 -> CmpEQ5/2
  Divide1/1 -> Convert1/1
  SufF6/1 -> CmpEQ1/2
  SufF7/1 -> CmpEQ4/2
  CmpEQ5/1 -> Or/5
  Convert1/1 -> Mult/2
  CmpEQ/1 -> And1/2
  Or/1 -> And1/1
  CmpEQ2/1 -> Or/1
  SFN/1 -> Sub/1, Divide1/1
  Sub/1 -> CmpEQ/2
  Mult/1 -> Sub/2
  SufF8/1 -> CmpEQ3/2
  Y/1 -> CmpEQ/1
  CmpEQ3/1 -> Or/4
  CmpEQ1/1 -> Or/2
  CmpEQ4/1 -> Or/3
  SufF9/1 -> CmpEQ2/2
  And1/1 -> Out2/1

== system Lib_LongPRACH/prach_wrap/S2B_FFT/S2B ==
  data_in : Inport
  data_valid : Inport  Port=2
  chin : Inport  Port=3
  ChannelIn : DSPBAPrim/ChannelIn  primtype=channelin  nInputs=dspba_internal_get_channel_ports(gcb)  nOutputs=dspba_internal_get_channel_ports(gcb)  omode=Inherit via internal rule  otype=sfix(16)  scale=2^-15  rndmethod=Unbiased  factor=1  satmethod=Symmetric  shift_vec=[0 1 2 -1]  value=1  inPortNames=['v'; 'c'; '0'; '1'; '2'; '3'; '4'; '5'; '6'; '7'; '8'; '9'; 'A'; 'B'; 'D'; 'E'; 'F'; 'G'; 'H'; 'I'; 'J'; 'K'; 'L'; 'M'; 'N'; 'O'; 'P'; 'Q'; 'R'; 'S'; 'T'; 'U'; 'W'; 'X'; 'Y'; 'Z']  outPortNames=['v'; 'c'; '0'; '1'; '2'; '3'; '4'; '5'; '6'; '7'; '8'; '9'; 'A'; 'B'; 'D'; 'E'; 'F'; 'G'; 'H'; 'I'; 'J'; 'K'; 'L'; 'M'; 'N'; 'O'; 'P'; 'Q'; 'R'; 'S'; 'T'; 'U'; 'W'; 'X'; 'Y'; 'Z']  dspbaimage=dspba_prim_channel_tall.svg  text=fprintf('In');  style=Optimised  dataSignals=1  foldingEnabled=off  channels=1  sampleRate=200  packetBeginPresent=off  packetBeginEnabled=off  visibilities=dspba_ChannelInVis(gcb)  latencyCorrection=0  scheduleOrigin=on  version=20211214
  ChannelOut : DSPBAPrim/ChannelOut  primtype=channelout  nInputs=dspba_internal_get_channel_ports(gcb)  nOutputs=dspba_internal_get_channel_ports(gcb)  omode=Inherit via internal rule  otype=sfix(16)  scale=2^-15  rndmethod=Unbiased  factor=1  satmethod=Symmetric  shift_vec=[0 1 2 -1]  value=1  inPortNames=['v'; 'c'; '0'; '1'; '2'; '3'; '4'; '5'; '6'; '7'; '8'; '9'; 'A'; 'B'; 'D'; 'E'; 'F'; 'G'; 'H'; 'I'; 'J'; 'K'; 'L'; 'M'; 'N'; 'O'; 'P'; 'Q'; 'R'; 'S'; 'T'; 'U'; 'W'; 'X'; 'Y'; 'Z']  outPortNames=['v'; 'c'; '0'; '1'; '2'; '3'; '4'; '5'; '6'; '7'; '8'; '9'; 'A'; 'B'; 'D'; 'E'; 'F'; 'G'; 'H'; 'I'; 'J'; 'K'; 'L'; 'M'; 'N'; 'O'; 'P'; 'Q'; 'R'; 'S'; 'T'; 'U'; 'W'; 'X'; 'Y'; 'Z']  dspbaimage=dspba_prim_channel_tall.svg  text=fprintf('Out%s', AdvDSPBChannelOutDisplay(latency));  style=Optimised  dataSignals=1  foldingEnabled=off  channels=1  sampleRate=200  packetBeginPresent=off  packetBeginEnabled=off  visibilities=dspba_ChannelOutVis(gcb)  latency=6  latencyCorrection=0  version=20211214
  DualMem : DSPBAPrim/DualMem  primtype=dualmem  nInputs=4  nOutputs=2  omode=Inherit via internal rule  otype=sfix(16)  scale=2^-15  rndmethod=Unbiased  factor=1  satmethod=Symmetric  shift_vec=[0 1 2 -1]  value=[zeros(1024*4*2, 1)]  inPortNames=['d1'; 'a1'; 'w1'; 'd2'; 'a2'; 'w2']  outPortNames=['q1'; 'q2']  dspbaimage=dspba_prim_tall.svg  text=fprintf('dmem%s',AdvDSPBDMemDisplay(UseDontCare));  style=Optimised  visibilities=8 + 1024 + 2^17 + 2^18  UseDontCare=on  TwinWritePorts=off  init=on  ProvideReadAccess=off  version=20211007
  S2B_control : Subsystem
  SynthesisInfo : DSPBAPrim/SynthesisInfo  primtype=synthinfo  nInputs=0  nOutputs=0  omode=Inherit via internal rule  otype=sfix(16)  scale=2^-15  rndmethod=Truncate  factor=1  satmethod=Symmetric  shift_vec=[0 1 2 -1]  value=99  inPortNames=[' '; ' ';]  outPortNames=[' ']  dspbaimage=dspba_prim_ctrl.jpg  text=fprintf('Style=%s', style);  style=Scheduled  visibilities=2^17+2^18+2^19+2^20+2^21+2^22+2^23+2^24  constraintPair=None  constraintRelation=>  constraintLimit=2  modelRefSign=+  modelRef=''  showSchedule=off  simulationMode=Use Global Value  resetMinimization=Conditional - On for ChannelIn/Out only  version=20220106
  Terminator : Terminator
  Terminator1 : Terminator
  data_out : Outport
  valid_out : Outport  Port=2
  ch_no : Outport  Port=3
  wires:
  S2B_control/2(We) -> DualMem/3
  S2B_control/1(Wr_addr_final) -> DualMem/2
  DualMem/1 -> Terminator/1
  S2B_control/3(rd_addr_final) -> DualMem/4
  S2B_control/5(ch_no) -> ChannelOut/2
  ChannelIn/3 -> DualMem/1
  data_in/1 -> ChannelIn/3
  ChannelIn/1 -> S2B_control/1(valid)
  data_valid/1 -> ChannelIn/1
  chin/1 -> ChannelIn/2
  ChannelIn/2 -> Terminator1/1
  ChannelOut/3 -> data_out/1
  DualMem/2 -> ChannelOut/3
  ChannelOut/1 -> valid_out/1
  S2B_control/4(rd_validout) -> ChannelOut/1
  ChannelOut/2 -> ch_no/1
